simulink model "local_oscilator_test_simulation_alone_v4"  (R2012b)
settings: Solver=ode45  StartTime=0.0  StopTime=100000  RelTol=1e-3
values from neighbouring files (symbols this model uses):
  Fs = 640e6    (= 640000000)    [filter_coefficients.m]    (also in filter_design.m; filter_design_getting_order.m)
undefined symbols (not defined in the file or in its folder): get, sided, Two
undefined symbols (not defined in the file): A_cos, A_sin, B_cos, B_sin, C_cos, C_sin, D_cos, D_sin
libraries: xbsIndex_r4 x394, dspsnks4 x10, dspsigops x4, simulink x2, casper_library_misc x1, xps_library x1
(part 1 of 5)
settings Model: Creator=heystek  LastModifiedBy=heystek

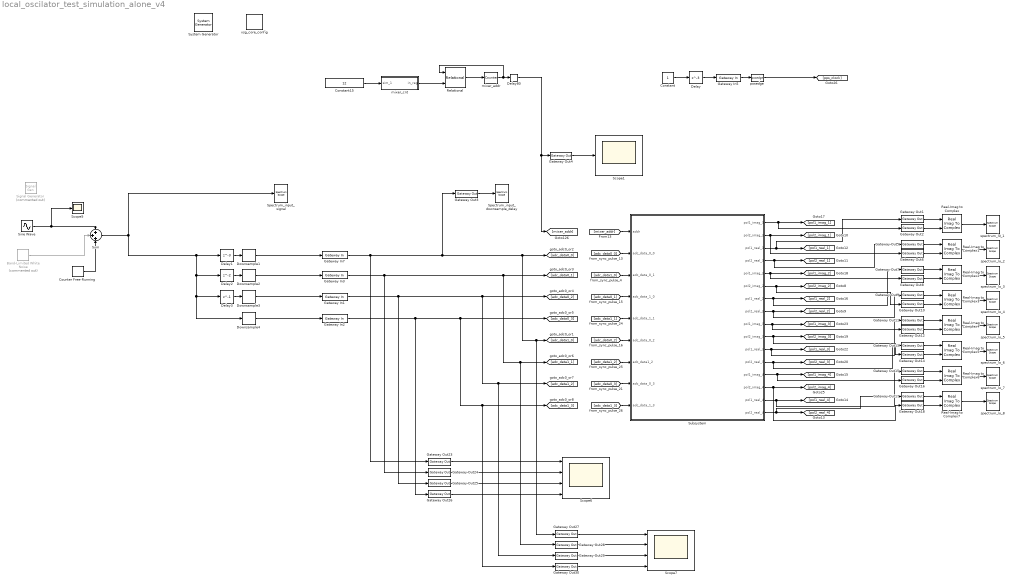
== system local_oscilator_test_simulation_alone_v4 ==
  " System Generator" : xbsIndex_r4/ System Generator  Tag=genX  xilinxfamily=virtex6  part=xc6vsx475t  speed=-1  package=ff1759  synthesis_tool=XST  clock_wrapper=Clock Enables  directory=./window_design/sysgen  proj_type=Project Navigator  Synth_file=XST Defaults  Impl_file=ISE Defaults  testbench=off  simulink_period=1  sysclk_period=6.25  dcm_input_clock_period=100  incr_netlist=off  trim_vbits=Everywhere in SubSystem  dbl_ovrd=According to Block Masks  core_generation=According to Block Masks  run_coregen=off  deprecated_control=off  eval_field=0  block_type=sysgen
  Band-Limited White Noise : simulink/Sources/Band-Limited White Noise  Commented=on  Cov=[0.01]  Ts=0.25  seed=[23341]
  Constant : Constant
  Constant15 : Constant  Value=12
  Counter Free-Running : simulink/Sources/Counter Free-Running  NumBits=8  tsamp=0.25
  Delay : Delay  DelayLength=3
  Delay1 : Delay  DelayLength=3
  Delay2 : Delay
  Delay3 : Delay  DelayLength=1
  Delay80 : xbsIndex_r4/Delay  rst=off  infoeditControl=Selection of Reset will increase slice count due to use of real FFs and instead of SRLs  en=off  latency=2  dbl_ovrd=off  reg_retiming=on  block_type=delay
      settings: block_version=11.4
  Downsample{1..4} (4 alike) : dspsigops/Downsample  N=4  phase=0  RateOptions=Enforce single-rate processing  smode=Allow multirate  fmode=Maintain input frame size  ic=0
  Gateway In{1..3,7} (4 alike) : xbsIndex_r4/Gateway In  gui_display_data_type=Fixed-point  arith_type="Signed  (2's comp)"  n_bits=16  bin_pt=15  preci_type=Single  exp_width=8  frac_width=24  quantization="Round  (unbiased: +/- Inf)"  overflow=Saturate  period=1  dbl_ovrd=off  timing_constraint=None  locs_specified=off  LOCs={}  UseAsADC=off  ADCChannel='1'  inherit_from_input=off  hdl_port=on  block_type=gatewayin
  Gateway In5 : xbsIndex_r4/Gateway In  gui_display_data_type=Boolean  arith_type=Boolean  n_bits=16  bin_pt=15  preci_type=Single  exp_width=8  frac_width=24  quantization="Round  (unbiased: +/- Inf)"  overflow=Saturate  period=1  dbl_ovrd=off  timing_constraint=None  locs_specified=off  LOCs={}  UseAsADC=off  ADCChannel='1'  inherit_from_input=off  hdl_port=on  block_type=gatewayin
  Gateway Out{1..18,23..29} (25 alike) : xbsIndex_r4/Gateway Out  inherit_from_input=on  hdl_port=on  timing_constraint=None  locs_specified=off  LOCs={}  UseAsDAC=off  DACChannel='1'  block_type=gatewayout
  Gateway Out30 : xbsIndex_r4/Gateway Out  inherit_from_input=off  hdl_port=on  timing_constraint=None  locs_specified=off  LOCs={}  UseAsDAC=off  DACChannel='1'  block_type=gatewayout
  Real-Imag to Complex{,1..7} (8 alike) : RealImagToComplex
  Relational : xbsIndex_r4/Relational  mode=a=b  en=off  latency=1  dbl_ovrd=off  block_type=relational
  Scope1 : Scope
      settings: SaveName=ScopeData7
  Scope5 : Scope
      settings: MaxDataPoints=10
  Scope6 : Scope  NumInputPorts=4
      settings: YMin=-5~-5~-5~-5  YMax=5~5~5~5
  Scope7 : Scope  NumInputPorts=4
      settings: YMin=-5~-5~-5~-5  YMax=5~5~5~5  SaveName=ScopeData2
  Signal Generator : SignalGenerator  Commented=on  Amplitude=0.1  Frequency=0.00353  VectorParams1D=off
  Sine Wave : Sin  SineType=Sample based  Amplitude=0.1  Frequency=5  Samples=2000  SampleTime=0.25  Offset=1
  Spectrum_input_downsample_delay : dspsnks4/Spectrum Scope  ScopeProperties=on  Domain=Frequency  HorizSpan=1  UseBuffer=on  BufferSize=2^13  Overlap=0  TreatMby1Signals=One channel  inpFftLenInherit=on  FFTlength=2^13  numAvg=5  DisplayProperties=off  AxisGrid=on  Memory=off  FrameNumber=on  AxisLegend=off  AxisZoom=off  OpenScopeAtSimStart=on  OpenScopeImmediately=off  FigPos=get(0,'defaultfigureposition')  AxisProperties=off  XUnits=Hertz  XRange=Two-sided ((-Fs/2...Fs/2])  XDisplay=0  InheritXIncr=on  XIncr=1.0  XLabel=Samples  XLimit=Auto  YUnits=dBW/Hertz  XMax=1  XMin=0  YLabel=Magnitude-squared, dB  LineProperties=off  wintypeSpecScope=Hann  RsSpecScope=50  betaSpecScope=5  winsampSpecScope=Periodic  XAxisParamsVer=6.9  isFrameUpgraded=on
      settings: YMin=-10  YMax=10
  Spectrum_input_signal : dspsnks4/Spectrum Scope  ScopeProperties=on  Domain=Frequency  HorizSpan=1  UseBuffer=on  BufferSize=2^15  Overlap=0  TreatMby1Signals=One channel  inpFftLenInherit=on  FFTlength=2^15  numAvg=1  DisplayProperties=off  AxisGrid=on  Memory=off  FrameNumber=on  AxisLegend=off  AxisZoom=off  OpenScopeAtSimStart=on  OpenScopeImmediately=off  FigPos=get(0,'defaultfigureposition')  AxisProperties=off  XUnits=Hertz  XRange=Two-sided ((-Fs/2...Fs/2])  XDisplay=0  InheritXIncr=on  XIncr=1.0  XLabel=Samples  XLimit=Auto  YUnits=dBW/Hertz  XMax=1  XMin=0  YLabel=Magnitude-squared, dB  LineProperties=off  wintypeSpecScope=Hann  RsSpecScope=50  betaSpecScope=5  winsampSpecScope=Periodic  XAxisParamsVer=6.9  isFrameUpgraded=on
      settings: YMin=-10  YMax=10
  Subsystem : Subsystem
  Sum : Sum  Inputs=+++
  mixer_addr : xbsIndex_r4/Counter  cnt_type=Free Running  cnt_to=Inf  operation=Up  start_count=0  cnt_by_val=1  arith_type=Unsigned  n_bits=16  bin_pt=0  load_pin=off  rst=on  en=off  explicit_period=on  period=1  dbl_ovrd=off  use_behavioral_HDL=off  implementation=Fabric  block_type=counter
      settings: block_version=11.4
  mixer_cnt : Subsystem  Tag=xps:sw_reg  AncestorBlock=xps_library/software_register  mask(swreg){io_dir=From Processor, io_delay=0, sample_period=1, names=reg, bitwidths=32, bin_pts=0, arith_types=0, sim_port=on, show_format=on}
      mask prompts: io_dir "I/O direction"; io_delay "I/O delay"; sample_period "Sample period"; names "Bitfield names [msb...lsb]"; bitwidths "Bitfield widths"; bin_pts "Bitfield binary pts"; arith_types "Bitfield types, ufix=0, fix=1, bool=2"; sim_port "Provide sim input/output?"; show_format "Print format string?"
      mask help: A 32-bit software-accessible register. Can be divided into bitfields of varying widths and types using the fields in the block mask.
      mask init:
      | try
      |     swreg_init(gcb)
      | catch ex
      |     disp(sprintf('%s: %s', gcb, ex.message))
      |     errordlg(ex.message)
      | end
      settings: AttributesFormatString=1input:uf32.0 = 32 bits
      mask TypeOptions io_dir: To Processor | From Processor
      mask Callback io_dir:
      | mask_enables = get_param(gcb, 'MaskEnables');
      | mask_names = get_param(gcb, 'MaskNames');
      | if strcmp(get_param(gcb, 'io_dir'), 'To Processor'),
      |     mask_enables{ismember(mask_names, 'sample_period')} = 'off';
      | else
      |     mask_enables{ismember(mask_names, 'sample_period')} = 'on';
      | end
      | set_param(gcb, 'MaskEnables', mask_enables);
  posedge : casper_library_misc/posedge  Tag=Rising Edge Detector
  spectrum_l0_1 : dspsnks4/Spectrum Scope  ScopeProperties=on  Domain=Frequency  HorizSpan=1  UseBuffer=on  BufferSize=2^13  Overlap=0  TreatMby1Signals=One channel  inpFftLenInherit=on  FFTlength=2^13  numAvg=5  DisplayProperties=off  AxisGrid=on  Memory=off  FrameNumber=on  AxisLegend=off  AxisZoom=off  OpenScopeAtSimStart=on  OpenScopeImmediately=off  FigPos=get(0,'defaultfigureposition')  AxisProperties=off  XUnits=Hertz  XRange=Two-sided ((-Fs/2...Fs/2])  XDisplay=0  InheritXIncr=on  XIncr=1.0  XLabel=Samples  XLimit=Auto  YUnits=dBW/Hertz  XMax=1  XMin=0  YLabel=Magnitude-squared, dB  LineProperties=off  wintypeSpecScope=Hann  RsSpecScope=50  betaSpecScope=5  winsampSpecScope=Periodic  XAxisParamsVer=6.9  isFrameUpgraded=on
      settings: YMin=-10  YMax=10
  spectrum_lo_2 : dspsnks4/Spectrum Scope  ScopeProperties=on  Domain=Frequency  HorizSpan=1  UseBuffer=on  BufferSize=2^13  Overlap=0  TreatMby1Signals=One channel  inpFftLenInherit=on  FFTlength=2^13  numAvg=5  DisplayProperties=off  AxisGrid=on  Memory=on  FrameNumber=on  AxisLegend=off  AxisZoom=off  OpenScopeAtSimStart=on  OpenScopeImmediately=off  FigPos=get(0,'defaultfigureposition')  AxisProperties=off  XUnits=Hertz  XRange=Two-sided ((-Fs/2...Fs/2])  XDisplay=0  InheritXIncr=on  XIncr=1.0  XLabel=Samples  XLimit=Auto  YUnits=dBW/Hertz  XMax=1  XMin=0  YLabel=Magnitude-squared, dB  LineProperties=off  wintypeSpecScope=Hann  RsSpecScope=50  betaSpecScope=5  winsampSpecScope=Periodic  XAxisParamsVer=6.9  isFrameUpgraded=on
      settings: YMin=-10  YMax=10
  spectrum_lo_{3..8} (6 alike) : dspsnks4/Spectrum Scope  ScopeProperties=on  Domain=Frequency  HorizSpan=1  UseBuffer=on  BufferSize=2^13  Overlap=0  TreatMby1Signals=One channel  inpFftLenInherit=on  FFTlength=2^13  numAvg=5  DisplayProperties=off  AxisGrid=on  Memory=off  FrameNumber=on  AxisLegend=off  AxisZoom=off  OpenScopeAtSimStart=on  OpenScopeImmediately=off  FigPos=get(0,'defaultfigureposition')  AxisProperties=off  XUnits=Hertz  XRange=Two-sided ((-Fs/2...Fs/2])  XDisplay=0  InheritXIncr=on  XIncr=1.0  XLabel=Samples  XLimit=Auto  YUnits=dBW/Hertz  XMax=1  XMin=0  YLabel=Magnitude-squared, dB  LineProperties=off  wintypeSpecScope=Hann  RsSpecScope=50  betaSpecScope=5  winsampSpecScope=Periodic  XAxisParamsVer=6.9  isFrameUpgraded=on
      settings: YMin=-10  YMax=10
  xsg_core_config : xps_library/XSG_core_config  Tag=xps:xsg  hw_sys=ROACH2:sx475t  clk_src=sys_clk  ROACH_clk_src=adc0_clk  ROACH2_clk_src=sys_clk  MKDIG_clk_src=sys_clk  clk_rate=200  sample_period=1  synthesis_tool=XST
  wires:
  Delay/1 -> Gateway In5/1
  Constant/1 -> Delay/1
  Gateway In5/1 -> posedge/1
  Downsample1/1 -> Gateway In7/1
  Band-Limited White Noise/1 -> Sum/2
  Sine Wave/1 -> Scope5/1, Sum/1
  Counter Free-Running/1 -> Sum/3
  Delay1/1 -> Downsample1/1
  Delay2/1 -> Downsample2/1
  Delay3/1 -> Downsample3/1
  posedge/1 -> [pps_clock]
  mixer_addr/1 -> Relational/1, Delay80/1
  Delay80/1 -> Gateway Out4/1, [mixer_addr]
  Relational/1 -> mixer_addr/1
  mixer_cnt/1(in_reg) -> Relational/2
  Constant15/1 -> mixer_cnt/1(sim_1)
  Subsystem/1(pol1_imag_1) -> Gateway Out2/1, [pol1_imag_1]
  Subsystem/2(pol2_imag_2) -> Gateway Out6/1, [pol2_imag_1]
  Subsystem/4(pol2_real_1) -> Gateway Out5/1, [pol2_real_1]
  Subsystem/5(pol1_imag_2) -> Gateway Out8/1, [pol1_imag_2]
  Subsystem/6("pol2_imag_2 ") -> Gateway Out10/1, [pol2_imag_2]
  Subsystem/7(pol1_real_2) -> Gateway Out7/1, [pol1_real_2]
  Subsystem/8(pol2_real_2) -> Gateway Out9/1, [pol2_real_2]
  Subsystem/9(pol1_imag_3) -> Gateway Out12/1, [pol1_imag_3]
  Subsystem/10(pol2_imag_3) -> Gateway Out14/1, [pol2_imag_3]
  Subsystem/11(pol1_real_3) -> Gateway Out11/1, [pol1_real_3]
  Subsystem/12(pol2_real_3) -> Gateway Out13/1, [pol2_real_3]
  Subsystem/13(pol1_imag_4) -> Gateway Out16/1, [pol1_imag_4]
  Subsystem/14(pol2_imag_4) -> Gateway Out18/1, [pol2_imag_4]
  Subsystem/15(pol1_real_4) -> Gateway Out15/1, [pol1_real_4]
  Subsystem/16(pol2_real_4) -> Gateway Out17/1, [pol2_real_4]
  [adc_data0_0] -> Subsystem/2(adc_data_0_0)
  [adc_data1_0] -> Subsystem/3(adc_data_0_1)
  [adc_data0_1] -> Subsystem/4(adc_data_1_0)
  [adc_data1_1] -> Subsystem/5(adc_data_1_1)
  [adc_data0_2] -> Subsystem/6(adc_data_0_2)
  [adc_data1_2] -> Subsystem/7(adc_data1_2)
  [adc_data0_3] -> Subsystem/8(adc_data_0_3)
  [adc_data1_3] -> Subsystem/9(adc_data_1_3)
  [mixer_addr] -> Subsystem/1(addr)
  Sum/1 -> Delay1/1, Delay2/1, Delay3/1, Downsample4/1, Spectrum_input_signal/1
  Downsample2/1 -> Gateway In3/1
  Downsample3/1 -> Gateway In1/1
  Downsample4/1 -> Gateway In2/1
  Gateway In7/1 -> Gateway Out23/1, Gateway Out3/1, Gateway Out27/1, [adc_data1_0], [adc_data0_0]
  Gateway In3/1 -> Gateway Out24/1, Gateway Out28/1, [adc_data1_1], [adc_data0_1]
  Gateway In2/1 -> Gateway Out26/1, Gateway Out30/1, [adc_data1_3], [adc_data0_3]
  Gateway Out3/1 -> Spectrum_input_downsample_delay/1
  Gateway Out23/1 -> Scope6/1
  Gateway Out24/1 -> Scope6/2
  Gateway Out25/1 -> Scope6/3
  Gateway Out26/1 -> Scope6/4
  Gateway In1/1 -> Gateway Out25/1, Gateway Out29/1, [adc_data1_2], [adc_data0_2]
  Gateway Out27/1 -> Scope7/1
  Gateway Out28/1 -> Scope7/2
  Gateway Out29/1 -> Scope7/3
  Gateway Out30/1 -> Scope7/4
  Subsystem/3(pol1_real_1) -> Gateway Out1/1, [pol1_real_1]
  Gateway Out4/1 -> Scope1/1
  Gateway Out1/1 -> Real-Imag to Complex/1
  Gateway Out2/1 -> Real-Imag to Complex/2
  Gateway Out5/1 -> Real-Imag to Complex1/1
  Gateway Out6/1 -> Real-Imag to Complex1/2
  Gateway Out7/1 -> Real-Imag to Complex2/1
  Gateway Out8/1 -> Real-Imag to Complex2/2
  Gateway Out9/1 -> Real-Imag to Complex3/1
  Gateway Out10/1 -> Real-Imag to Complex3/2
  Gateway Out11/1 -> Real-Imag to Complex4/1
  Gateway Out12/1 -> Real-Imag to Complex4/2
  Gateway Out13/1 -> Real-Imag to Complex5/1
  Gateway Out14/1 -> Real-Imag to Complex5/2
  Gateway Out15/1 -> Real-Imag to Complex6/1
  Gateway Out16/1 -> Real-Imag to Complex6/2
  Gateway Out17/1 -> Real-Imag to Complex7/1
  Gateway Out18/1 -> Real-Imag to Complex7/2
  Real-Imag to Complex/1 -> spectrum_l0_1/1
  Real-Imag to Complex7/1 -> spectrum_lo_8/1
  Real-Imag to Complex6/1 -> spectrum_lo_7/1
  Real-Imag to Complex5/1 -> spectrum_lo_6/1
  Real-Imag to Complex4/1 -> spectrum_lo_5/1
  Real-Imag to Complex3/1 -> spectrum_lo_4/1
  Real-Imag to Complex2/1 -> spectrum_lo_3/1
  Real-Imag to Complex1/1 -> spectrum_lo_2/1

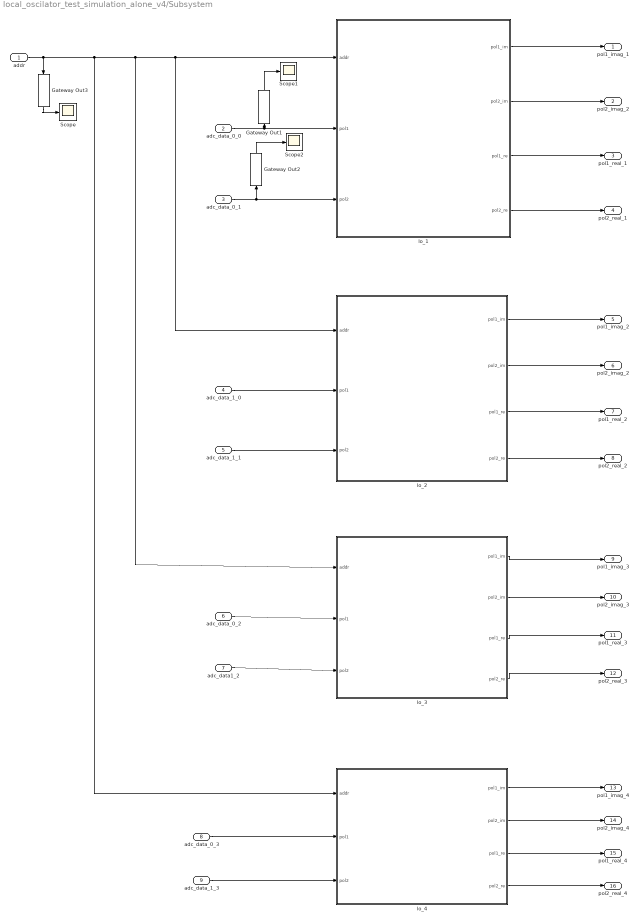
== system local_oscilator_test_simulation_alone_v4/Subsystem ==
  addr : Inport
  adc_data_0_0 : Inport  Port=2
  adc_data_0_1 : Inport  Port=3
  adc_data_1_0 : Inport  Port=4
  adc_data_1_1 : Inport  Port=5
  adc_data_0_2 : Inport  Port=6
  adc_data1_2 : Inport  Port=7
  adc_data_0_3 : Inport  Port=8
  adc_data_1_3 : Inport  Port=9
  Gateway Out1 : xbsIndex_r4/Gateway Out  inherit_from_input=on  hdl_port=on  timing_constraint=None  locs_specified=off  LOCs={}  UseAsDAC=off  DACChannel='1'  block_type=gatewayout
  Gateway Out2 : xbsIndex_r4/Gateway Out  inherit_from_input=on  hdl_port=on  timing_constraint=None  locs_specified=off  LOCs={}  UseAsDAC=off  DACChannel='1'  block_type=gatewayout
  Gateway Out3 : xbsIndex_r4/Gateway Out  inherit_from_input=on  hdl_port=on  timing_constraint=None  locs_specified=off  LOCs={}  UseAsDAC=off  DACChannel='1'  block_type=gatewayout
  Scope : Scope
      settings: SaveName=ScopeData4
  Scope1 : Scope
      settings: YMin=-0.11  YMax=0.11  SaveName=ScopeData5
  Scope2 : Scope
      settings: YMin=-0.11  YMax=0.11  SaveName=ScopeData6
  lo_1 : Subsystem  AncestorBlock=gbt_library/complex_mix_lo
  lo_2 : Subsystem  AncestorBlock=gbt_library/complex_mix_lo
  lo_3 : Subsystem  AncestorBlock=gbt_library/complex_mix_lo
  lo_4 : Subsystem  AncestorBlock=gbt_library/complex_mix_lo
  pol1_imag_1 : Outport
  pol2_imag_2 : Outport  Port=2
  pol1_real_1 : Outport  Port=3
  pol2_real_1 : Outport  Port=4
  pol1_imag_2 : Outport  Port=5
  "pol2_imag_2 " : Outport  Port=6
  pol1_real_2 : Outport  Port=7
  pol2_real_2 : Outport  Port=8
  pol1_imag_3 : Outport  Port=9
  pol2_imag_3 : Outport  Port=10
  pol1_real_3 : Outport  Port=11
  pol2_real_3 : Outport  Port=12
  pol1_imag_4 : Outport  Port=13
  pol2_imag_4 : Outport  Port=14
  pol1_real_4 : Outport  Port=15
  pol2_real_4 : Outport  Port=16
  wires:
  lo_1/3(pol1_re) -> pol1_real_1/1
  lo_4/4(pol2_re) -> pol2_real_4/1
  adc_data_0_1/1 -> lo_1/3(pol2), Gateway Out2/1
  adc_data_1_0/1 -> lo_2/2(pol1)
  lo_4/3(pol1_re) -> pol1_real_4/1
  lo_4/2(pol2_im) -> pol2_imag_4/1
  adc_data_0_3/1 -> lo_4/2(pol1)
  lo_3/4(pol2_re) -> pol2_real_3/1
  adc_data_1_3/1 -> lo_4/3(pol2)
  lo_1/1(pol1_im) -> pol1_imag_1/1
  adc_data1_2/1 -> lo_3/3(pol2)
  lo_2/1(pol1_im) -> pol1_imag_2/1
  lo_1/4(pol2_re) -> pol2_real_1/1
  lo_2/3(pol1_re) -> pol1_real_2/1
  adc_data_0_0/1 -> lo_1/2(pol1), Gateway Out1/1
  lo_1/2(pol2_im) -> pol2_imag_2/1
  lo_4/1(pol1_im) -> pol1_imag_4/1
  adc_data_0_2/1 -> lo_3/2(pol1)
  lo_3/3(pol1_re) -> pol1_real_3/1
  adc_data_1_1/1 -> lo_2/3(pol2)
  lo_2/4(pol2_re) -> pol2_real_2/1
  addr/1 -> Gateway Out3/1, lo_4/1(addr), lo_2/1(addr), lo_1/1(addr), lo_3/1(addr)
  lo_3/1(pol1_im) -> pol1_imag_3/1
  lo_3/2(pol2_im) -> pol2_imag_3/1
  lo_2/2(pol2_im) -> "pol2_imag_2 "/1
  Gateway Out3/1 -> Scope/1
  Gateway Out1/1 -> Scope1/1
  Gateway Out2/1 -> Scope2/1

== system local_oscilator_test_simulation_alone_v4/mixer_cnt ==
  sim_1 : Inport
  io_delay : xbsIndex_r4/Delay  rst=off  infoeditControl=Selection of Reset will increase slice count due to use of real FFs and instead of SRLs  en=off  latency=0  dbl_ovrd=off  reg_retiming=on  block_type=delay
  local_oscilator_test_simulation_alone_v4_mixer_cnt_user_data_out : xbsIndex_r4/Gateway In  gui_display_data_type=Fixed-point  arith_type=Unsigned  n_bits=32  bin_pt=0  preci_type=Single  exp_width=8  frac_width=24  quantization="Round  (unbiased: +/- Inf)"  overflow=Saturate  period=1  dbl_ovrd=off  timing_constraint=None  locs_specified=off  LOCs={}  UseAsADC=off  ADCChannel='1'  inherit_from_input=off  hdl_port=on  block_type=gatewayin
  reint1 : xbsIndex_r4/Reinterpret  force_arith_type=on  arith_type=Unsigned  force_bin_pt=on  bin_pt=0  block_type=reinterpret
  slice_reg : xbsIndex_r4/Slice  nbits=32  boolean_output=off  mode=Lower Bit Location + Width  bit1=0  base1=MSB of Input  bit0=0  base0=LSB of Input  dbl_ovrd=off  block_type=slice
  in_reg : Outport
  wires:
  local_oscilator_test_simulation_alone_v4_mixer_cnt_user_data_out/1 -> io_delay/1
  sim_1/1 -> local_oscilator_test_simulation_alone_v4_mixer_cnt_user_data_out/1
  io_delay/1 -> slice_reg/1
  slice_reg/1 -> reint1/1
  reint1/1 -> in_reg/1

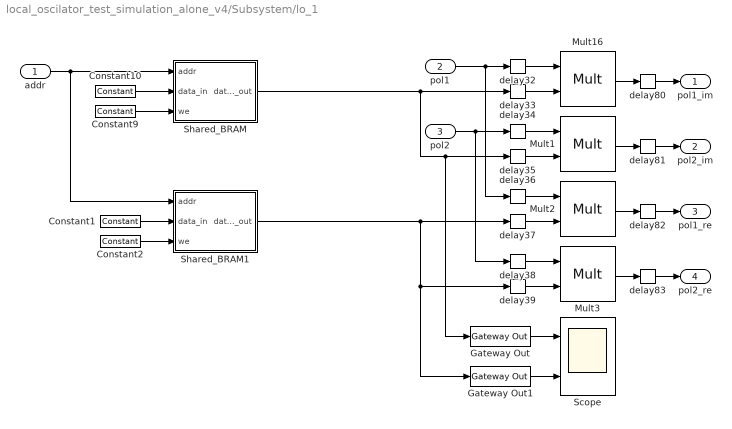
== system local_oscilator_test_simulation_alone_v4/Subsystem/lo_1 ==
  addr : Inport
  pol1 : Inport  Port=2
  pol2 : Inport  Port=3
  Constant{1..2,9..10} (4 alike) : xbsIndex_r4/Constant  const=0  gui_display_data_type=Fixed-point  arith_type=Unsigned  n_bits=18  bin_pt=0  preci_type=Single  exp_width=8  frac_width=24  explicit_period=on  period=1  equ=P=C  opselect=C  inp2=PCIN>>17  opr=+  inp1=P  carry=CIN  dbl_ovrd=off  block_type=constant
  Gateway Out : xbsIndex_r4/Gateway Out  inherit_from_input=off  hdl_port=on  timing_constraint=None  locs_specified=off  LOCs={}  UseAsDAC=off  DACChannel='1'  block_type=gatewayout
      settings: infoedit="Gateway out block.  Converts Xilinx fixed point or floating-point type inputs into ouputs of type Simulink integer, double, or fixed point.<br><br>Hardware notes:  In hardware these blocks become top level output ports or are discarded, depending on how they are configured."
  Gateway Out1 : xbsIndex_r4/Gateway Out  inherit_from_input=off  hdl_port=on  timing_constraint=None  locs_specified=off  LOCs={}  UseAsDAC=off  DACChannel='1'  block_type=gatewayout
      settings: infoedit="Gateway out block.  Converts Xilinx fixed point or floating-point type inputs into ouputs of type Simulink integer, double, or fixed point.<br><br>Hardware notes:  In hardware these blocks become top level output ports or are discarded, depending on how they are configured."
  Mult{1..3,16} (4 alike) : xbsIndex_r4/Mult  precision=User Defined  arith_type="Signed  (2's comp)"  n_bits=16  bin_pt=15  quantization=Truncate  overflow=Wrap  en=off  latency=5  dbl_ovrd=off  use_behavioral_HDL=off  opt=Speed  use_embedded=on  optimum_pipeline=off  pipeline=on  use_rpm=on  placement_style=Triangular  block_type=mult
      settings: block_version=11.4
  Scope : Scope  NumInputPorts=2
      settings: YMin=-0.0075~-1  YMax=0.0075~1  SaveName=ScopeData3
  Shared_BRAM : Subsystem  Tag=xps:bram  AncestorBlock=xps_library/Shared_BRAM  mask{arith_type=Signed  (2's comp), addr_width=10, data_width=32, reg_prim_output=off, reg_core_output=off, optimization=Minimum_Area, data_bin_pt=0, init_vals=A_sin, sample_rate=1}
      mask prompts: arith_type "Output Data Type"; addr_width "Address width"; data_width "Data Width"; reg_prim_output "Register Primitive Output"; reg_core_output "Register Core Output"; data_bin_pt "Data Binary Point"; init_vals "Initial values (simulation only)"; sample_rate "Sample rate"
      mask init:
      | shared_bram_mask;
      mask TypeOptions arith_type: Unsigned | Signed  (2's comp)
      mask TypeOptions data_width: 8 | 16 | 32 | 64 | 128
      mask TypeOptions optimization: Minimum_Area | Low_Power
  Shared_BRAM1 : Subsystem  Tag=xps:bram  AncestorBlock=xps_library/Shared_BRAM  mask{arith_type=Signed  (2's comp), addr_width=10, data_width=32, reg_prim_output=off, reg_core_output=off, optimization=Minimum_Area, data_bin_pt=0, init_vals=A_cos, sample_rate=1}
      mask prompts: arith_type "Output Data Type"; addr_width "Address width"; data_width "Data Width"; reg_prim_output "Register Primitive Output"; reg_core_output "Register Core Output"; data_bin_pt "Data Binary Point"; init_vals "Initial values (simulation only)"; sample_rate "Sample rate"
      mask init:
      | shared_bram_mask;
      mask TypeOptions arith_type: Unsigned | Signed  (2's comp)
      mask TypeOptions data_width: 8 | 16 | 32 | 64 | 128
      mask TypeOptions optimization: Minimum_Area | Low_Power
  delay{32..39,80..83} (12 alike) : xbsIndex_r4/Delay  rst=off  infoeditControl=Selection of Reset will increase slice count due to use of real FFs and instead of SRLs  en=off  latency=1  dbl_ovrd=off  reg_retiming=on  block_type=delay
      settings: block_version=11.4
  pol1_im : Outport
  pol2_im : Outport  Port=2
  pol1_re : Outport  Port=3
  pol2_re : Outport  Port=4
  wires:
  Constant9/1 -> Shared_BRAM/3(we)
  Constant10/1 -> Shared_BRAM/2(data_in)
  Mult16/1 -> delay80/1
  Shared_BRAM/1(data_out) -> delay33/1, delay35/1, Gateway Out/1
  Mult1/1 -> delay81/1
  Mult2/1 -> delay82/1
  Shared_BRAM1/1(data_out) -> delay37/1, delay39/1, Gateway Out1/1
  Mult3/1 -> delay83/1
  delay32/1 -> Mult16/1
  delay33/1 -> Mult16/2
  delay34/1 -> Mult1/1
  delay35/1 -> Mult1/2
  delay36/1 -> Mult2/1
  delay37/1 -> Mult2/2
  delay38/1 -> Mult3/1
  delay39/1 -> Mult3/2
  delay80/1 -> pol1_im/1
  pol2/1 -> delay34/1, delay38/1
  delay81/1 -> pol2_im/1
  delay82/1 -> pol1_re/1
  delay83/1 -> pol2_re/1
  pol1/1 -> delay32/1, delay36/1
  Gateway Out/1 -> Scope/1
  Gateway Out1/1 -> Scope/2
  Constant2/1 -> Shared_BRAM1/3(we)
  Constant1/1 -> Shared_BRAM1/2(data_in)
  addr/1 -> Shared_BRAM1/1(addr), Shared_BRAM/1(addr)

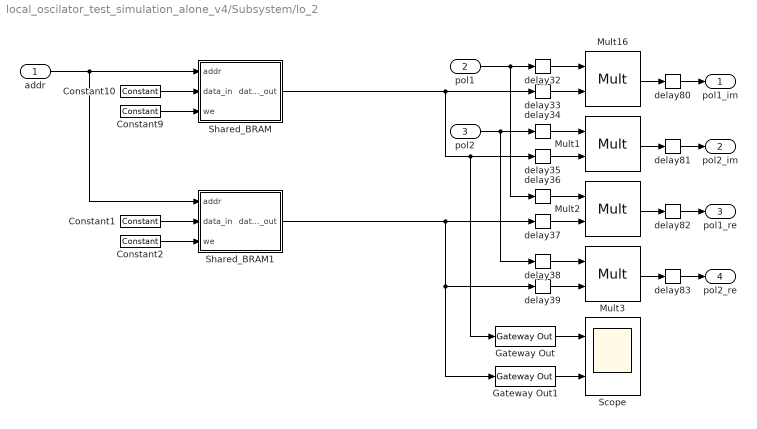
== system local_oscilator_test_simulation_alone_v4/Subsystem/lo_2 ==
  addr : Inport
  pol1 : Inport  Port=2
  pol2 : Inport  Port=3
  Constant{1..2,9..10} (4 alike) : xbsIndex_r4/Constant  const=0  gui_display_data_type=Fixed-point  arith_type=Unsigned  n_bits=18  bin_pt=0  preci_type=Single  exp_width=8  frac_width=24  explicit_period=on  period=1  equ=P=C  opselect=C  inp2=PCIN>>17  opr=+  inp1=P  carry=CIN  dbl_ovrd=off  block_type=constant
  Gateway Out : xbsIndex_r4/Gateway Out  inherit_from_input=off  hdl_port=on  timing_constraint=None  locs_specified=off  LOCs={}  UseAsDAC=off  DACChannel='1'  block_type=gatewayout
      settings: infoedit="Gateway out block.  Converts Xilinx fixed point or floating-point type inputs into ouputs of type Simulink integer, double, or fixed point.<br><br>Hardware notes:  In hardware these blocks become top level output ports or are discarded, depending on how they are configured."
  Gateway Out1 : xbsIndex_r4/Gateway Out  inherit_from_input=off  hdl_port=on  timing_constraint=None  locs_specified=off  LOCs={}  UseAsDAC=off  DACChannel='1'  block_type=gatewayout
      settings: infoedit="Gateway out block.  Converts Xilinx fixed point or floating-point type inputs into ouputs of type Simulink integer, double, or fixed point.<br><br>Hardware notes:  In hardware these blocks become top level output ports or are discarded, depending on how they are configured."
  Mult{1..3,16} (4 alike) : xbsIndex_r4/Mult  precision=User Defined  arith_type="Signed  (2's comp)"  n_bits=16  bin_pt=15  quantization=Truncate  overflow=Wrap  en=off  latency=5  dbl_ovrd=off  use_behavioral_HDL=off  opt=Speed  use_embedded=on  optimum_pipeline=off  pipeline=on  use_rpm=on  placement_style=Triangular  block_type=mult
      settings: block_version=11.4
  Scope : Scope  NumInputPorts=2
      settings: YMin=-0.0075~-1  YMax=0.0075~1  SaveName=ScopeData3
  Shared_BRAM : Subsystem  Tag=xps:bram  AncestorBlock=xps_library/Shared_BRAM  mask{arith_type=Signed  (2's comp), addr_width=10, data_width=32, reg_prim_output=off, reg_core_output=off, optimization=Minimum_Area, data_bin_pt=0, init_vals=B_sin, sample_rate=1}
      mask prompts: arith_type "Output Data Type"; addr_width "Address width"; data_width "Data Width"; reg_prim_output "Register Primitive Output"; reg_core_output "Register Core Output"; data_bin_pt "Data Binary Point"; init_vals "Initial values (simulation only)"; sample_rate "Sample rate"
      mask init:
      | shared_bram_mask;
      mask TypeOptions arith_type: Unsigned | Signed  (2's comp)
      mask TypeOptions data_width: 8 | 16 | 32 | 64 | 128
      mask TypeOptions optimization: Minimum_Area | Low_Power
  Shared_BRAM1 : Subsystem  Tag=xps:bram  AncestorBlock=xps_library/Shared_BRAM  mask{arith_type=Signed  (2's comp), addr_width=10, data_width=32, reg_prim_output=off, reg_core_output=off, optimization=Minimum_Area, data_bin_pt=0, init_vals=B_cos, sample_rate=1}
      mask prompts: arith_type "Output Data Type"; addr_width "Address width"; data_width "Data Width"; reg_prim_output "Register Primitive Output"; reg_core_output "Register Core Output"; data_bin_pt "Data Binary Point"; init_vals "Initial values (simulation only)"; sample_rate "Sample rate"
      mask init:
      | shared_bram_mask;
      mask TypeOptions arith_type: Unsigned | Signed  (2's comp)
      mask TypeOptions data_width: 8 | 16 | 32 | 64 | 128
      mask TypeOptions optimization: Minimum_Area | Low_Power
  delay{32..39,80..83} (12 alike) : xbsIndex_r4/Delay  rst=off  infoeditControl=Selection of Reset will increase slice count due to use of real FFs and instead of SRLs  en=off  latency=1  dbl_ovrd=off  reg_retiming=on  block_type=delay
      settings: block_version=11.4
  pol1_im : Outport
  pol2_im : Outport  Port=2
  pol1_re : Outport  Port=3
  pol2_re : Outport  Port=4
  wires:
  Constant9/1 -> Shared_BRAM/3(we)
  Constant10/1 -> Shared_BRAM/2(data_in)
  Mult16/1 -> delay80/1
  Shared_BRAM/1(data_out) -> delay33/1, delay35/1, Gateway Out/1
  Mult1/1 -> delay81/1
  Mult2/1 -> delay82/1
  Shared_BRAM1/1(data_out) -> delay37/1, delay39/1, Gateway Out1/1
  Mult3/1 -> delay83/1
  delay32/1 -> Mult16/1
  delay33/1 -> Mult16/2
  delay34/1 -> Mult1/1
  delay35/1 -> Mult1/2
  delay36/1 -> Mult2/1
  delay37/1 -> Mult2/2
  delay38/1 -> Mult3/1
  delay39/1 -> Mult3/2
  delay80/1 -> pol1_im/1
  pol2/1 -> delay34/1, delay38/1
  delay81/1 -> pol2_im/1
  delay82/1 -> pol1_re/1
  delay83/1 -> pol2_re/1
  pol1/1 -> delay32/1, delay36/1
  addr/1 -> Shared_BRAM1/1(addr), Shared_BRAM/1(addr)
  Gateway Out/1 -> Scope/1
  Gateway Out1/1 -> Scope/2
  Constant1/1 -> Shared_BRAM1/2(data_in)
  Constant2/1 -> Shared_BRAM1/3(we)

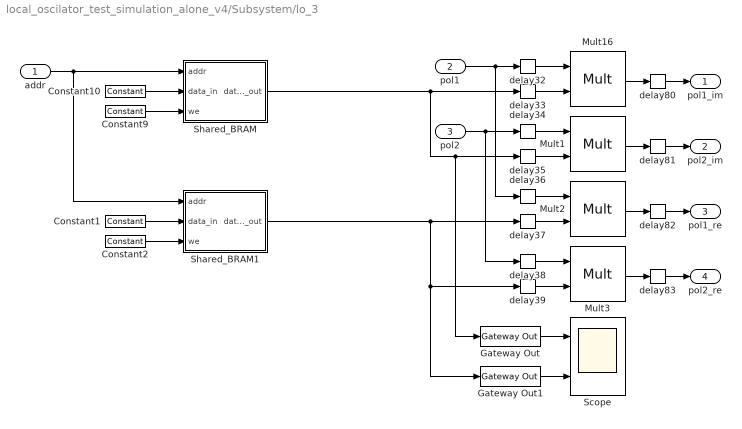
== system local_oscilator_test_simulation_alone_v4/Subsystem/lo_3 ==
  addr : Inport
  pol1 : Inport  Port=2
  pol2 : Inport  Port=3
  Constant{1..2,9..10} (4 alike) : xbsIndex_r4/Constant  const=0  gui_display_data_type=Fixed-point  arith_type=Unsigned  n_bits=18  bin_pt=0  preci_type=Single  exp_width=8  frac_width=24  explicit_period=on  period=1  equ=P=C  opselect=C  inp2=PCIN>>17  opr=+  inp1=P  carry=CIN  dbl_ovrd=off  block_type=constant
  Gateway Out : xbsIndex_r4/Gateway Out  inherit_from_input=off  hdl_port=on  timing_constraint=None  locs_specified=off  LOCs={}  UseAsDAC=off  DACChannel='1'  block_type=gatewayout
      settings: infoedit="Gateway out block.  Converts Xilinx fixed point or floating-point type inputs into ouputs of type Simulink integer, double, or fixed point.<br><br>Hardware notes:  In hardware these blocks become top level output ports or are discarded, depending on how they are configured."
  Gateway Out1 : xbsIndex_r4/Gateway Out  inherit_from_input=off  hdl_port=on  timing_constraint=None  locs_specified=off  LOCs={}  UseAsDAC=off  DACChannel='1'  block_type=gatewayout
      settings: infoedit="Gateway out block.  Converts Xilinx fixed point or floating-point type inputs into ouputs of type Simulink integer, double, or fixed point.<br><br>Hardware notes:  In hardware these blocks become top level output ports or are discarded, depending on how they are configured."
  Mult{1..3,16} (4 alike) : xbsIndex_r4/Mult  precision=User Defined  arith_type="Signed  (2's comp)"  n_bits=16  bin_pt=15  quantization=Truncate  overflow=Wrap  en=off  latency=5  dbl_ovrd=off  use_behavioral_HDL=off  opt=Speed  use_embedded=on  optimum_pipeline=off  pipeline=on  use_rpm=on  placement_style=Triangular  block_type=mult
      settings: block_version=11.4
  Scope : Scope  NumInputPorts=2
      settings: YMin=-0.0075~-1  YMax=0.0075~1  SaveName=ScopeData3
  Shared_BRAM : Subsystem  Tag=xps:bram  AncestorBlock=xps_library/Shared_BRAM  mask{arith_type=Signed  (2's comp), addr_width=10, data_width=32, reg_prim_output=off, reg_core_output=off, optimization=Minimum_Area, data_bin_pt=0, init_vals=C_sin, sample_rate=1}
      mask prompts: arith_type "Output Data Type"; addr_width "Address width"; data_width "Data Width"; reg_prim_output "Register Primitive Output"; reg_core_output "Register Core Output"; data_bin_pt "Data Binary Point"; init_vals "Initial values (simulation only)"; sample_rate "Sample rate"
      mask init:
      | shared_bram_mask;
      mask TypeOptions arith_type: Unsigned | Signed  (2's comp)
      mask TypeOptions data_width: 8 | 16 | 32 | 64 | 128
      mask TypeOptions optimization: Minimum_Area | Low_Power
  Shared_BRAM1 : Subsystem  Tag=xps:bram  AncestorBlock=xps_library/Shared_BRAM  mask{arith_type=Signed  (2's comp), addr_width=10, data_width=32, reg_prim_output=off, reg_core_output=off, optimization=Minimum_Area, data_bin_pt=0, init_vals=C_cos, sample_rate=1}
      mask prompts: arith_type "Output Data Type"; addr_width "Address width"; data_width "Data Width"; reg_prim_output "Register Primitive Output"; reg_core_output "Register Core Output"; data_bin_pt "Data Binary Point"; init_vals "Initial values (simulation only)"; sample_rate "Sample rate"
      mask init:
      | shared_bram_mask;
      mask TypeOptions arith_type: Unsigned | Signed  (2's comp)
      mask TypeOptions data_width: 8 | 16 | 32 | 64 | 128
      mask TypeOptions optimization: Minimum_Area | Low_Power
  delay{32..39,80..83} (12 alike) : xbsIndex_r4/Delay  rst=off  infoeditControl=Selection of Reset will increase slice count due to use of real FFs and instead of SRLs  en=off  latency=1  dbl_ovrd=off  reg_retiming=on  block_type=delay
      settings: block_version=11.4
  pol1_im : Outport
  pol2_im : Outport  Port=2
  pol1_re : Outport  Port=3
  pol2_re : Outport  Port=4
  wires:
  Constant9/1 -> Shared_BRAM/3(we)
  Constant10/1 -> Shared_BRAM/2(data_in)
  Mult16/1 -> delay80/1
  Shared_BRAM/1(data_out) -> delay33/1, delay35/1, Gateway Out/1
  Mult1/1 -> delay81/1
  Mult2/1 -> delay82/1
  Shared_BRAM1/1(data_out) -> delay37/1, delay39/1, Gateway Out1/1
  Mult3/1 -> delay83/1
  delay32/1 -> Mult16/1
  delay33/1 -> Mult16/2
  delay34/1 -> Mult1/1
  delay35/1 -> Mult1/2
  delay36/1 -> Mult2/1
  delay37/1 -> Mult2/2
  delay38/1 -> Mult3/1
  delay39/1 -> Mult3/2
  delay80/1 -> pol1_im/1
  pol2/1 -> delay34/1, delay38/1
  delay81/1 -> pol2_im/1
  delay82/1 -> pol1_re/1
  delay83/1 -> pol2_re/1
  pol1/1 -> delay32/1, delay36/1
  addr/1 -> Shared_BRAM1/1(addr), Shared_BRAM/1(addr)
  Gateway Out/1 -> Scope/1
  Gateway Out1/1 -> Scope/2
  Constant2/1 -> Shared_BRAM1/3(we)
  Constant1/1 -> Shared_BRAM1/2(data_in)

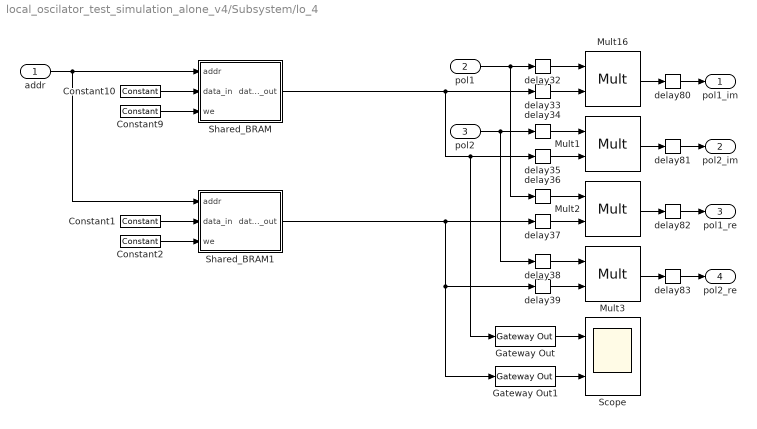
== system local_oscilator_test_simulation_alone_v4/Subsystem/lo_4 ==
  addr : Inport
  pol1 : Inport  Port=2
  pol2 : Inport  Port=3
  Constant{1..2,9..10} (4 alike) : xbsIndex_r4/Constant  const=0  gui_display_data_type=Fixed-point  arith_type=Unsigned  n_bits=18  bin_pt=0  preci_type=Single  exp_width=8  frac_width=24  explicit_period=on  period=1  equ=P=C  opselect=C  inp2=PCIN>>17  opr=+  inp1=P  carry=CIN  dbl_ovrd=off  block_type=constant
  Gateway Out : xbsIndex_r4/Gateway Out  inherit_from_input=off  hdl_port=on  timing_constraint=None  locs_specified=off  LOCs={}  UseAsDAC=off  DACChannel='1'  block_type=gatewayout
      settings: infoedit="Gateway out block.  Converts Xilinx fixed point or floating-point type inputs into ouputs of type Simulink integer, double, or fixed point.<br><br>Hardware notes:  In hardware these blocks become top level output ports or are discarded, depending on how they are configured."
  Gateway Out1 : xbsIndex_r4/Gateway Out  inherit_from_input=off  hdl_port=on  timing_constraint=None  locs_specified=off  LOCs={}  UseAsDAC=off  DACChannel='1'  block_type=gatewayout
      settings: infoedit="Gateway out block.  Converts Xilinx fixed point or floating-point type inputs into ouputs of type Simulink integer, double, or fixed point.<br><br>Hardware notes:  In hardware these blocks become top level output ports or are discarded, depending on how they are configured."
  Mult{1..3,16} (4 alike) : xbsIndex_r4/Mult  precision=User Defined  arith_type="Signed  (2's comp)"  n_bits=16  bin_pt=15  quantization=Truncate  overflow=Wrap  en=off  latency=5  dbl_ovrd=off  use_behavioral_HDL=off  opt=Speed  use_embedded=on  optimum_pipeline=off  pipeline=on  use_rpm=on  placement_style=Triangular  block_type=mult
      settings: block_version=11.4
  Scope : Scope  NumInputPorts=2
      settings: YMin=-0.0075~-1  YMax=0.0075~1  SaveName=ScopeData3
  Shared_BRAM : Subsystem  Tag=xps:bram  AncestorBlock=xps_library/Shared_BRAM  mask{arith_type=Signed  (2's comp), addr_width=10, data_width=32, reg_prim_output=off, reg_core_output=off, optimization=Minimum_Area, data_bin_pt=0, init_vals=D_sin, sample_rate=1}
      mask prompts: arith_type "Output Data Type"; addr_width "Address width"; data_width "Data Width"; reg_prim_output "Register Primitive Output"; reg_core_output "Register Core Output"; data_bin_pt "Data Binary Point"; init_vals "Initial values (simulation only)"; sample_rate "Sample rate"
      mask init:
      | shared_bram_mask;
      mask TypeOptions arith_type: Unsigned | Signed  (2's comp)
      mask TypeOptions data_width: 8 | 16 | 32 | 64 | 128
      mask TypeOptions optimization: Minimum_Area | Low_Power
  Shared_BRAM1 : Subsystem  Tag=xps:bram  AncestorBlock=xps_library/Shared_BRAM  mask{arith_type=Signed  (2's comp), addr_width=10, data_width=32, reg_prim_output=off, reg_core_output=off, optimization=Minimum_Area, data_bin_pt=0, init_vals=D_cos, sample_rate=1}
      mask prompts: arith_type "Output Data Type"; addr_width "Address width"; data_width "Data Width"; reg_prim_output "Register Primitive Output"; reg_core_output "Register Core Output"; data_bin_pt "Data Binary Point"; init_vals "Initial values (simulation only)"; sample_rate "Sample rate"
      mask init:
      | shared_bram_mask;
      mask TypeOptions arith_type: Unsigned | Signed  (2's comp)
      mask TypeOptions data_width: 8 | 16 | 32 | 64 | 128
      mask TypeOptions optimization: Minimum_Area | Low_Power
  delay{32..39,80..83} (12 alike) : xbsIndex_r4/Delay  rst=off  infoeditControl=Selection of Reset will increase slice count due to use of real FFs and instead of SRLs  en=off  latency=1  dbl_ovrd=off  reg_retiming=on  block_type=delay
      settings: block_version=11.4
  pol1_im : Outport
  pol2_im : Outport  Port=2
  pol1_re : Outport  Port=3
  pol2_re : Outport  Port=4
  wires:
  Constant9/1 -> Shared_BRAM/3(we)
  Constant10/1 -> Shared_BRAM/2(data_in)
  Mult16/1 -> delay80/1
  Shared_BRAM/1(data_out) -> delay33/1, delay35/1, Gateway Out/1
  Mult1/1 -> delay81/1
  Mult2/1 -> delay82/1
  Shared_BRAM1/1(data_out) -> delay37/1, delay39/1, Gateway Out1/1
  Mult3/1 -> delay83/1
  delay32/1 -> Mult16/1
  delay33/1 -> Mult16/2
  delay34/1 -> Mult1/1
  delay35/1 -> Mult1/2
  delay36/1 -> Mult2/1
  delay37/1 -> Mult2/2
  delay38/1 -> Mult3/1
  delay39/1 -> Mult3/2
  delay80/1 -> pol1_im/1
  pol2/1 -> delay34/1, delay38/1
  delay81/1 -> pol2_im/1
  delay82/1 -> pol1_re/1
  delay83/1 -> pol2_re/1
  pol1/1 -> delay32/1, delay36/1
  addr/1 -> Shared_BRAM1/1(addr), Shared_BRAM/1(addr)
  Gateway Out/1 -> Scope/1
  Gateway Out1/1 -> Scope/2
  Constant2/1 -> Shared_BRAM1/3(we)
  Constant1/1 -> Shared_BRAM1/2(data_in)

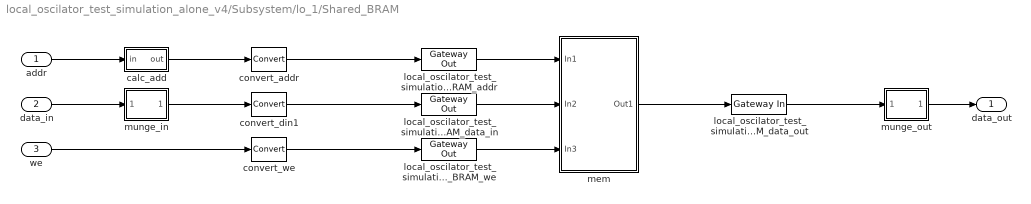
== system local_oscilator_test_simulation_alone_v4/Subsystem/lo_1/Shared_BRAM ==
  addr : Inport
  data_in : Inport  Port=2
  we : Inport  Port=3
  calc_add : Subsystem  mask{data_width=32, addr_width=10, sample_rate=sample_rate}
      mask prompts: data_width "data width"; addr_width "address width"; sample_rate "sample rate"
  convert_addr : xbsIndex_r4/Convert  gui_display_data_type=Fixed-point  arith_type=Unsigned  n_bits=addr_width  bin_pt=0  float_type=Single  exp_bits=8  fraction_bits=24  quantization=Truncate  overflow=Wrap  en=off  latency=0  dbl_ovrd=off  pipeline=off  block_type=convert
      settings: xl_area=[0, 0, 0, 0, 0, 0, 0]
  convert_din1 : xbsIndex_r4/Convert  gui_display_data_type=Fixed-point  arith_type=Unsigned  n_bits=32  bin_pt=0  float_type=Single  exp_bits=8  fraction_bits=24  quantization=Truncate  overflow=Wrap  en=off  latency=0  dbl_ovrd=off  pipeline=off  block_type=convert
      settings: xl_area=[0, 0, 0, 0, 0, 0, 0]
  convert_we : xbsIndex_r4/Convert  gui_display_data_type=Fixed-point  arith_type=Unsigned  n_bits=1  bin_pt=0  float_type=Single  exp_bits=8  fraction_bits=24  quantization=Truncate  overflow=Wrap  en=off  latency=0  dbl_ovrd=off  pipeline=off  block_type=convert
      settings: xl_area=[0, 0, 0, 0, 0, 0, 0]
  local_oscilator_test_simulation_alone_v4_Subsystem_lo_1_Shared_BRAM_addr : xbsIndex_r4/Gateway Out  inherit_from_input=off  hdl_port=on  timing_constraint=None  locs_specified=off  LOCs={'A5','B9','A9','C1','A3','G6','E9','A6','A7','A8','B8','B1','B3','D9','B5','B4','B6','C2'}  UseAsDAC=off  DACChannel='1'  block_type=gatewayout
      settings: infoedit="Gateway out block.  Converts Xilinx fixed point inputs into ouputs of type Simulink integer, double, or fixed point.<P><P>Hardware notes:  In hardware these blocks become top level output ports or are discarded, depending on how they are configured."  xl_area=[0, 0, 0, 0, 0, 0, 0]  sginterface={'Nallatech'=>{'xdspkit'=>{'non_memory_mapped_port'=>'uprev_Shared_BRAM_addr'}},'Xilinx'=>{'jtaghwcosim'=>{'non_memory_mapped_port'=>'uprev_Shared_BRAM_addr'},'xdspkit'=>{'non_memory_mapped_port'=>'uprev_Shared_BRAM_addr'}}}
  local_oscilator_test_simulation_alone_v4_Subsystem_lo_1_Shared_BRAM_data_in : xbsIndex_r4/Gateway Out  inherit_from_input=off  hdl_port=on  timing_constraint=None  locs_specified=off  LOCs={'B21','B22','A22','B23','B19','C19','A20','A21','A23','B24','A24','A25','E18','D18','C18','B18'}  UseAsDAC=off  DACChannel='1'  block_type=gatewayout
      settings: infoedit="Gateway out block.  Converts Xilinx fixed point inputs into ouputs of type Simulink integer, double, or fixed point.<P><P>Hardware notes:  In hardware these blocks become top level output ports or are discarded, depending on how they are configured."  xl_area=[0, 0, 0, 0, 0, 0, 0]  sginterface={'Nallatech'=>{'xdspkit'=>{'non_memory_mapped_port'=>'uprev_Shared_BRAM_data_in'}},'Xilinx'=>{'jtaghwcosim'=>{'non_memory_mapped_port'=>'uprev_Shared_BRAM_data_in'},'xdspkit'=>{'non_memory_mapped_port'=>'uprev_Shared_BRAM_data_in'}}}
  local_oscilator_test_simulation_alone_v4_Subsystem_lo_1_Shared_BRAM_data_out : xbsIndex_r4/Gateway In  gui_display_data_type=Fixed-point  arith_type=Unsigned  n_bits=32  bin_pt=0  preci_type=Single  exp_width=8  frac_width=24  quantization=Truncate  overflow=Wrap  period=sample_rate  dbl_ovrd=off  timing_constraint=None  locs_specified=off  LOCs={}  UseAsADC=off  ADCChannel='1'  inherit_from_input=off  hdl_port=on  block_type=gatewayin
      settings: xl_area=[0, 0, 0, 0, 0, 0, 0]
  local_oscilator_test_simulation_alone_v4_Subsystem_lo_1_Shared_BRAM_we : xbsIndex_r4/Gateway Out  inherit_from_input=off  hdl_port=on  timing_constraint=None  locs_specified=off  LOCs={'A14'}  UseAsDAC=off  DACChannel='1'  block_type=gatewayout
      settings: infoedit="Gateway out block.  Converts Xilinx fixed point inputs into ouputs of type Simulink integer, double, or fixed point.<P><P>Hardware notes:  In hardware these blocks become top level output ports or are discarded, depending on how they are configured."  xl_area=[0, 0, 0, 0, 0, 0, 0]
  mem : Subsystem
  munge_in : Subsystem  AncestorBlock=casper_library_flow_control/munge  mask(munge){divisions=1, div_size=32, order=[0], arith_type_out=Unsigned, bin_pt_out=0}
      mask prompts: divisions "Number of divisions"; div_size "Division size (bits)"; order "Division packing order"; arith_type_out "Output arithmetic type"; bin_pt_out "Output binary point"
      mask help: Splits an input bus into the specified number of divisions and then recombines them in the order specified (most significant division = 0,least = number divisions-1)
      mask init:
      | munge_init(gcb, ...
      |     'divisions', divisions, ...
      |     'div_size', div_size, ...
      |     'order', order, ...
      |     'arith_type_out', arith_type_out, ...
      |     'bin_pt_out', bin_pt_out);
      settings: AttributesFormatString=|
      | split:32
      | join:0
      | Unsigned [32,0]
      mask TypeOptions arith_type_out: Unsigned | Signed  (2's comp) | Floating-point
  munge_out : Subsystem  AncestorBlock=casper_library_flow_control/munge  mask(munge){divisions=1, div_size=32, order=[0], arith_type_out=Signed  (2's comp), bin_pt_out=0}
      mask prompts: divisions "Number of divisions"; div_size "Division size (bits)"; order "Division packing order"; arith_type_out "Output arithmetic type"; bin_pt_out "Output binary point"
      mask help: Splits an input bus into the specified number of divisions and then recombines them in the order specified (most significant division = 0,least = number divisions-1)
      mask init:
      | munge_init(gcb, ...
      |     'divisions', divisions, ...
      |     'div_size', div_size, ...
      |     'order', order, ...
      |     'arith_type_out', arith_type_out, ...
      |     'bin_pt_out', bin_pt_out);
      settings: AttributesFormatString=|
      | split:32
      | join:0
      | Signed  (2's comp) [32,0]
      mask TypeOptions arith_type_out: Unsigned | Signed  (2's comp) | Floating-point
  data_out : Outport
  wires:
  convert_addr/1 -> local_oscilator_test_simulation_alone_v4_Subsystem_lo_1_Shared_BRAM_addr/1
  convert_din1/1 -> local_oscilator_test_simulation_alone_v4_Subsystem_lo_1_Shared_BRAM_data_in/1
  data_in/1 -> munge_in/1(din)
  calc_add/1(out) -> convert_addr/1
  local_oscilator_test_simulation_alone_v4_Subsystem_lo_1_Shared_BRAM_we/1 -> mem/3(In3)
  local_oscilator_test_simulation_alone_v4_Subsystem_lo_1_Shared_BRAM_data_in/1 -> mem/2(In2)
  local_oscilator_test_simulation_alone_v4_Subsystem_lo_1_Shared_BRAM_addr/1 -> mem/1(In1)
  convert_we/1 -> local_oscilator_test_simulation_alone_v4_Subsystem_lo_1_Shared_BRAM_we/1
  local_oscilator_test_simulation_alone_v4_Subsystem_lo_1_Shared_BRAM_data_out/1 -> munge_out/1(din)
  mem/1(Out1) -> local_oscilator_test_simulation_alone_v4_Subsystem_lo_1_Shared_BRAM_data_out/1
  addr/1 -> calc_add/1(in)
  we/1 -> convert_we/1
  munge_out/1(dout) -> data_out/1
  munge_in/1(dout) -> convert_din1/1
